simulink model "HybridSMC_NN_Abbasi_22_01_2022_MM_2014a"  (Simulink 10.0)
settings: Solver=ode45  StartTime=0.0  StopTime=10  RelTol=1e-3  EnableMultiTasking=on
settings Model: Creator=SBU  LastModifiedBy=Abbasi
settings DataIOCC: LimitDataPoints=on  SaveFormat=StructureWithTime
settings DebuggingCC: UnderspecifiedInitializationDetection=Simplified  MergeDetectMultiDrivingBlocksExec=error
settings HardwareCC: ProdBitPerPointer=64  ProdLargestAtomicFloat=Float  ProdIntDivRoundTo=Zero  ProdEndianess=LittleEndian  ProdHWDeviceType=Specified
settings GRTTargetCC: CombineOutputUpdateFcns=on  GRTInterface=off
settings ConfigComp: CovExternalEMLEnable=off

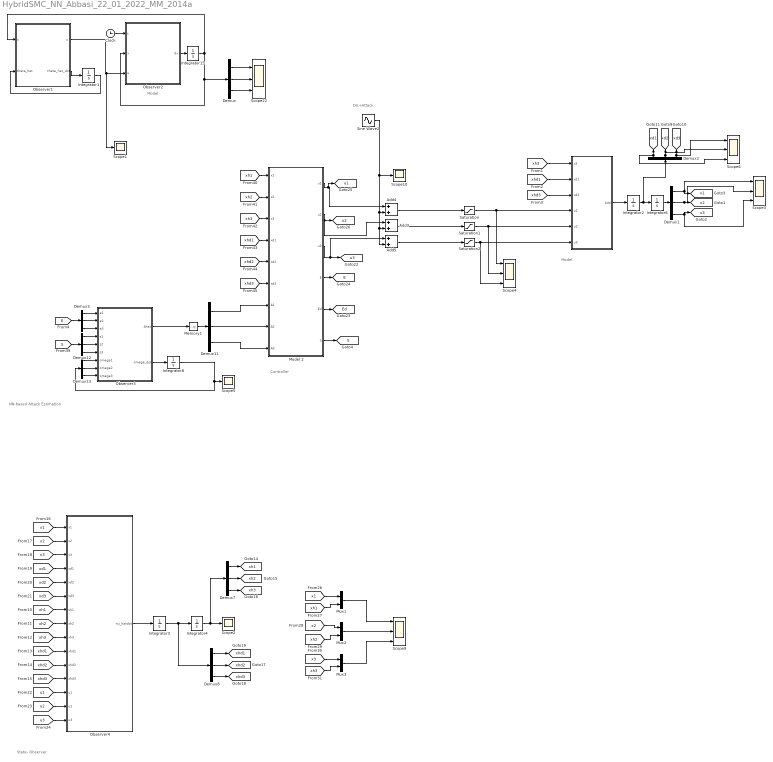
== system HybridSMC_NN_Abbasi_22_01_2022_MM_2014a ==
  note: Model
  note: Dis+Attack
  note: State- Observer
  note: NN-based Attack Estimation
  note: Controller
  note: Model
  " " : MATLAB Function  TreatAsAtomicUnit=on
  Add3 : Sum
  Add4 : Sum
  Add5 : Sum
  Clock : Clock
  Demux{,1..3,7..8,11..13} (9 alike) : Demux  Outputs=3
  Integrator1 : Integrator  InitialCondition=0.001*ones(27,1)  UpperSaturationLimit=0.1  LowerSaturationLimit=-0.1
  Integrator15 : Integrator  InitialCondition=[0.3;-0.3;-0.4]  UpperSaturationLimit=0.5  LowerSaturationLimit=-0.5
  Integrator2 : Integrator  InitialCondition=[0;0;0]  UpperSaturationLimit=0.1  LowerSaturationLimit=-0.1
  Integrator3 : Integrator  InitialCondition=[0;0;0]  LimitOutput=on  UpperSaturationLimit=500  LowerSaturationLimit=-500
  Integrator4 : Integrator  InitialCondition=[2;0.5;1.5]  UpperSaturationLimit=10  LowerSaturationLimit=-10
  Integrator6 : Integrator  InitialCondition=[3;1;1]  UpperSaturationLimit=10  LowerSaturationLimit=-10
  Integrator8 : Integrator  InitialCondition=0.1*[0.1;0.1;0.1]
  Memory1 : Memory
  Model 2 : MATLAB Function  TreatAsAtomicUnit=on
  Mux1 : Mux  Inputs=2
  Mux2 : Mux  Inputs=2
  Mux3 : Mux  Inputs=2
  Observer1 : MATLAB Function  TreatAsAtomicUnit=on
  Observer2 : MATLAB Function  TreatAsAtomicUnit=on
  Observer3 : MATLAB Function  TreatAsAtomicUnit=on
  Observer4 : MATLAB Function  TreatAsAtomicUnit=on
  Saturation : Saturate  UpperLimit=100  LowerLimit=-100
  Saturation1 : Saturate  UpperLimit=100  LowerLimit=-100
  Saturation2 : Saturate  UpperLimit=100  LowerLimit=-100
  Scope{1..2,5,10} (4 alike) : Scope
  Scope{3..4,6,9,22} (5 alike) : Scope  NumInputPorts=3
  Sine Wave2 : Sin  Amplitude=0.8  Bias=0.5  Frequency=2*pi  SampleTime=0
  tag scope: E=global, Ed=global, S=global, u1=global, u2=global, u3=global, x1=global, x2=global, x3=global, xd1=global, xd2=global, xd3=global, xh1=global, xh2=global, xh3=global, xhd1=global, xhd2=global, xhd3=global
  wires:
  Observer2/1(dx) -> Integrator15/1
  Integrator15/1 -> Observer1/1(x), Observer2/2(x), Demux/1
  Clock/1 -> Observer2/1(t)
  Observer1/2(theta_hat_dot) -> Integrator1/1
  Integrator1/1 -> Observer1/2(theta_hat)
  Observer1/1(u) -> Scope1/1, Observer2/3(u)
  Demux/1 -> Scope22/1
  Demux/2 -> Scope22/2
  Demux/3 -> Scope22/3
  Model 2/3(u3) -> Add5/1, [u3]
  [xh1] -> Model 2/1(x1)
  [xh2] -> Model 2/2(x2)
  [xh3] -> Model 2/3(x3)
  [xhd1] -> Model 2/4(xd1)
  [xhd2] -> Model 2/5(xd2)
  [xhd3] -> Model 2/6(xd3)
  Observer3/2(omega_dot) -> Integrator8/1
  Observer3/1(Ahat) -> Memory1/1
  Model 2/4(E) -> [E]
  [S] -> Demux12/1
  Demux12/1 -> Observer3/4(s1)
  Demux11/2 -> Model 2/8(A2)
  Demux11/3 -> Model 2/9(A3)
  Model 2/2(u2) -> Add3/1, [u2]
  Add3/1 -> Saturation1/1
  Model 2/1(u1) -> [u1], Add4/1
  Add4/1 -> Saturation/1
  Demux11/1 -> Model 2/7(A1)
  Add5/1 -> Saturation2/1
  Sine Wave2/1 -> Add4/2, Add3/2, Add5/2, Scope10/1
  Model 2/5(Ed) -> [Ed]
  " "/1(Xdd) -> Integrator2/1
  Integrator2/1 -> Demux2/1, Integrator6/1
  Integrator6/1 -> Demux1/1
  Demux1/1 -> Scope3/1, [x1]
  Demux1/2 -> Scope3/2, [x2]
  Demux1/3 -> Scope3/3, [x3]
  Demux2/1 -> Scope6/3, [xd1]
  Demux2/2 -> Scope6/2, [xd2]
  [xh3] -> " "/1(x3)
  [xhd1] -> " "/2(xd1)
  [xhd3] -> " "/3(xd3)
  Saturation/1 -> " "/4(u1), Scope4/1
  Saturation1/1 -> " "/5(u2), Scope4/2
  Saturation2/1 -> " "/6(u3), Scope4/3
  Model 2/6(S) -> [S]
  Demux12/2 -> Observer3/5(s2)
  Demux12/3 -> Observer3/6(s3)
  Demux13/1 -> Observer3/7(omega1)
  Demux13/2 -> Observer3/8(omega2)
  Demux13/3 -> Observer3/9(omega3)
  [E] -> Demux3/1
  Demux3/1 -> Observer3/1(e1)
  Demux3/2 -> Observer3/2(e2)
  Demux3/3 -> Observer3/3(e3)
  Memory1/1 -> Demux11/1
  Integrator8/1 -> Scope5/1, Demux13/1
  Observer4/1(nu_hatdot) -> Integrator3/1
  Integrator4/1 -> Demux7/1, Scope2/1
  Demux7/1 -> [xh1]
  Demux7/2 -> [xh2]
  Demux7/3 -> [xh3]
  Integrator3/1 -> Integrator4/1, Demux8/1
  Demux8/1 -> [xhd1]
  Demux8/2 -> [xhd2]
  Demux8/3 -> [xhd3]
  [xhd3] -> Observer4/12(xhd3)
  [xhd2] -> Observer4/11(xhd2)
  [xhd1] -> Observer4/10(xhd1)
  [xh3] -> Observer4/9(xh3)
  [xh2] -> Observer4/8(xh2)
  [xh1] -> Observer4/7(xh1)
  [x1] -> Observer4/1(x1)
  [x2] -> Observer4/2(x2)
  [x3] -> Observer4/3(x3)
  [xd1] -> Observer4/4(xd1)
  [xd2] -> Observer4/5(xd2)
  [xd3] -> Observer4/6(xd3)
  [u1] -> Observer4/13(u1)
  [u2] -> Observer4/14(u2)
  [u3] -> Observer4/15(u3)
  [x1] -> Mux1/1
  [xh1] -> Mux1/2
  [x2] -> Mux2/1
  [xh2] -> Mux2/2
  Mux2/1 -> Scope9/2
  [x3] -> Mux3/1
  [xh3] -> Mux3/2
  Mux3/1 -> Scope9/3
  Mux1/1 -> Scope9/1
  Demux2/3 -> Scope6/1, [xd3]

== matlab function Observer1 ==
  data: x input double; u output double; theta_hat input double; theta_hat_dot output double
function  [u,theta_hat_dot] = fcn(x,theta_hat)

x1=x(1);
x2=x(2);
x3=x(3);

gt = 1;
kt = 1;
s = 1;
m = 27;
fb = 0.8;

pmax = 120.185;
tb = sqrt(m)*fb/(2*pmax);

ka1 = 1.5; ka2 = 2; ku = 2.5;
mu = [-0.6 0 0.6]';
% u = zeros (length(t),1);


    phii = exp(-norm(x'-mu')^2/(2*s^2));
    phi = phii*ones(27,1);
    pt = theta_hat.*phi;
    z1 = x1;
    a1 = -ka1 * z1;
    z2 = x2 - a1;
   a2 = -(ka1 + ka2)*z2 + z1*ka1^2;
    z3 = x3-a2;
    
    a2dot = -ka1^3*z1 + (ka1^2 + ka1*ka2 + ka2^2)*z2 - (ka1+ka2)*z3;
    zeta = 1e-6;
    db = 0.1;
    
    u = -ku*z3 - tanh(z3*pt/zeta)'*pt - tanh(z3*a2dot/zeta)*a2dot - tanh(z3*fb/(2*zeta))*fb/2-tanh(z3*db/zeta)*db;

    
  
   
ck = 0;
 for j = 1:27
     if theta_hat(j) == 0
         ck = 1;
     end
 end
         
         
    
if ((norm(theta_hat) == tb) && (z3 > 0))||((z3<0)&&(ck == 1))
     theta_hat_dot = zeros(27,1);
 else
     theta_hat_dot = gt*(z3*phi-kt*theta_hat);
end
end

== matlab function Observer3 ==
  data: e1 input double; e2 input double; e3 input double; s1 input double; s2 input double; s3 input double; Ahat output double; omega_dot output double; omega1 input double; omega2 input double; omega3 input double
function [Ahat,omega_dot] = fcn( e1,e2,e3,s1,s2,s3,omega1,omega2,omega3)

Sigma = 1.5; 
G1 = exp(-norm(e1)^2/2*Sigma^2);
OmgaDot1 = -s1 * G1;
Ahat1 = omega1'*G1;

G2 = exp(-norm(e2)^2/2*Sigma^2);
OmgaDot2 = -s2 * G2;
Ahat2 = omega2'*G2;

G3 = exp(-norm(e3)^2/2*Sigma^2);
OmgaDot3 = -s3 * G3;
Ahat3 = omega3'*G3;

Ahat = [Ahat1 Ahat2 Ahat3]';
omega_dot = [OmgaDot1 OmgaDot2 OmgaDot3]';

== matlab function Observer4 ==
  data: x1 input double; x2 input double; x3 input double; nu_hatdot output double; xd1 input double; xd2 input double; xd3 input double; xh1 input double; xh2 input double; xh3 input double; xhd1 input double; xhd2 input double; xhd3 input double; u1 input double; u2 input double; u3 input double

function nu_hatdot  = fcn(x1,x2,x3,xd1,xd2,xd3,xh1,xh2,xh3,xhd1,xhd2,xhd3,u1,u2,u3)

landa1 = 10.5; 
landa2 = 10.5;
landa3 = 10.5;

e1 = x1 -xh1;
ed1 = xd1 - xhd1;
s1 = ed1 + landa1*e1;
e2 = x2 -xh2;
ed2 = xd2 - xhd2;
s2 = ed2 + landa2*e2;
e3 = x3 -xh3;
ed3 = xd3 - xhd3;
s3 = ed3 + landa3*e3;

a1 = 20; a2 = 40; y1 = 0.5; y2 = 2.5;

m1 = 3; 
m2 = 1; 
J = 5; 
g = 9.81;


G1 = a1*abs(s1)^y1*sign(s1)+a2*abs(s1)^y2*sign(s1);
G2 = a1*abs(s2)^y1*sign(s2)+a2*abs(s2)^y2*sign(s2);
G3 = a1*abs(s3)^y1*sign(s3)+a2*abs(s3)^y2*sign(s3);


nu_hatdot1 = 2*(m2/J)*x3*xd1*xd3 + (1/J)*u1 + G1; 
nu_hatdot2 = g*x3 + (1/(m1+m2))*u2 + G2; 
nu_hatdot3 = m2*x3*xd1^2 + (1/m2)*u3 + G3; 

nu_hatdot = [nu_hatdot1, nu_hatdot2, nu_hatdot3]';

== matlab function   ==
  data: x3 input double; Xdd output double; xd1 input double; xd3 input double; u1 input double; u2 input double; u3 input double

function Xdd = fcn(x3,xd1,xd3,u1,u2,u3)
m1 = 3; 
m2 = 1; 
J = 5; 
g = 9.81;
f = [2*(m2/J)*x3*xd1*xd3;g*x3;-m2*x3*xd1^2];
g = [(1/J)*u1;u2/(m1+m2);(1/m2)*u3];

Xdd = f + g;

== matlab function Model 2 ==
  data: x1 input double; x2 input double; x3 input double; xd1 input double; xd2 input double; xd3 input double; u1 output double; u2 output double; u3 output double; A1 input double; A2 input double; A3 input double; E output double; Ed output double; S output double

function [u1,u2,u3,E,Ed,S] = fcn(x1,x2,x3,xd1,xd2,xd3,A1,A2,A3)
% [x1_dot,x2_dot,x3_dot,x4_dot,x5_dot,x6_dot] = fcn(x3,x4,x5,x6,u1,u2,u3)
m1 = 3; 
m2 = 1; 
J = 5; 
g = 9.81;

x1_d = 0;
x2_d = 0; 
x3_d = 0; 
xd1_d = 0; 
xd2_d = 0; 
xd3_d = 0; 
x_dd1 = 0;
x_dd2 = 0; 
x_dd3 = 0; 

% landa = 1.5;

landa1 = 7.5; 
landa2 = 5.5;
landa3 = 5.5;
K1 = 10.5; K2 = 10.1; K3 = 10.1;

a1 = 10; a2 = 20; y1 = 0.5; y2 = 2.5;

e1 = x1 - x1_d;
ed1 = xd1 - xd1_d;
s1 = ed1 + landa1*e1;
e2 = x2 - x2_d;
ed2 = xd2 - xd2_d;
s2 = ed2 + landa2*e2;
e3 = x3 - x3_d;
ed3 = xd3 - xd3_d;
s3 = ed3 + landa3*e3;

E = [e1 e2 e3]';
Ed = [ed1 ed2 ed3]';

N1 = (-a1*abs(s1)^y1*sign(s1)-a2*abs(s1)^y2*sign(s1));
N2 = (-a1*abs(s2)^y1*sign(s2)-a2*abs(s2)^y2*sign(s2));
N3 = (-a1*abs(s3)^y1*sign(s3)-a2*abs(s3)^y2*sign(s3));

% u1 = (1/(1/J))*(-2*(m2/J)*x3*xd1*xd3+x_dd1-landa1*ed1-A1)+(-K1*tanh(s1));
% u2 = (m1+m2)*(-g*x3+x_dd2-landa2*ed2-A2)+(-K2*tanh(s2));
% u3 = (m2)*(m2*x3*xd1^2+x_dd3-landa3*ed3-A3)+(-K3*tanh(s3));
u1 = (1/(1/J))*(-2*(m2/J)*x3*xd1*xd3+x_dd1-landa1*ed1-A1)+(-K1*tanh(s1)+N1);
u2 = (m1+m2)*(-g*x3+x_dd2-landa2*ed2-A2)+(-K2*tanh(s2)+N2);
u3 = (m2)*(m2*x3*xd1^2+x_dd3-landa3*ed3-A3)+(-K3*tanh(s3)+N3);
S = [s1 s2 s3]';

% N = (-K3*tanh(s3)-a1*abs(s3)^y1*sign(s3)-a2*abs(s3)^y2*sign(s3));

== matlab function Observer2 ==
  data: t input double; x input double; dx output double; u input double
function dx = Model(t,x,u)
x1dot = x(2);
x2dot = x(3);
x3dot = (x(1)^2*x(3)^2 + x(2)^4) + (x(1)^2 + 2*sin(x(2))+3)*u + 0.1*sin(t)*sin(0.1*t);
dx = [x1dot x2dot x3dot]';
end
